simulink model "autonomy1_first_run"  (R2018a)
settings: Solver=VariableStepAuto  StartTime=0.0  StopTime=inf  RelTol=1e-3
InitFcn:
  | run('initArena.m')
undefined symbols (not defined in the file): allObstacles, endPt, wall
settings Model: SnapshotBufferSize=20  SnapshotInterval=1  Creator=alex  LastModifiedBy=alex

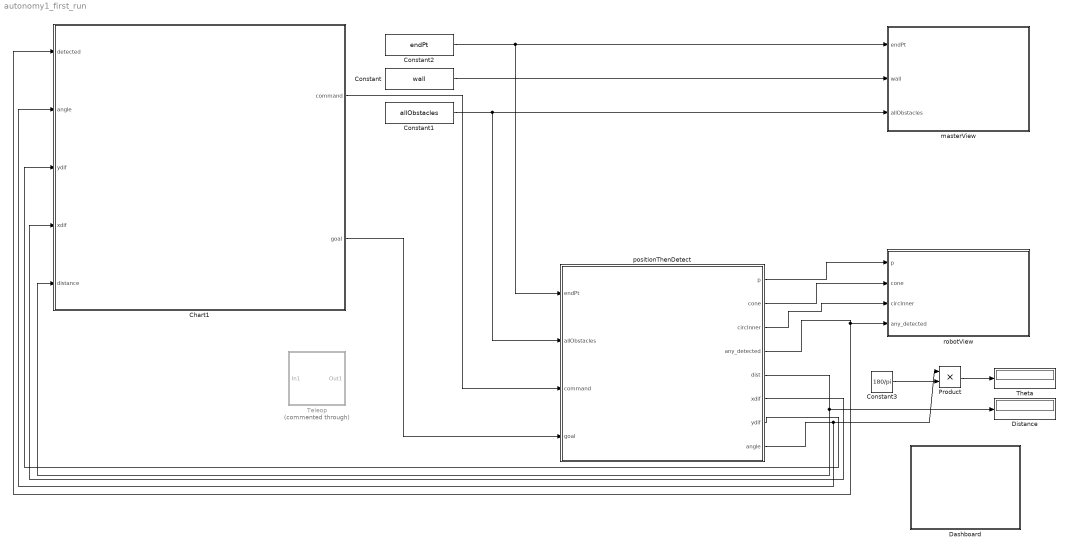
== system autonomy1_first_run ==
  Chart1 : Stateflow chart  TreatAsAtomicUnit=on
  Constant : Constant  Value=wall
  Constant1 : Constant  Value=allObstacles
  Constant2 : Constant  Value=endPt
  Constant3 : Constant  Value=180/pi
  Dashboard : Subsystem
  "Distance " : Display
  Product : Product
  "Teleop " : Subsystem  Commented=through
  Theta : Display
  masterView : MATLAB Function  TreatAsAtomicUnit=on
  positionThenDetect : MATLAB Function  TreatAsAtomicUnit=on
  robotView : MATLAB Function  TreatAsAtomicUnit=on
  wires:
  Constant/1 -> masterView/2(wall)
  Constant1/1 -> positionThenDetect/2(allObstacles), masterView/3(allObstacles)
  Chart1/1(command) -> positionThenDetect/3(command)
  positionThenDetect/4(any_detected) -> robotView/4(any_detected), Chart1/1(detected)
  Constant2/1 -> positionThenDetect/1(endPt), masterView/1(endPt)
  Constant3/1 -> Product/2
  positionThenDetect/8(angle) -> Chart1/2(angle), Product/1
  Product/1 -> Theta/1
  positionThenDetect/5(dist) -> Chart1/5(distance), "Distance "/1
  positionThenDetect/6(xdif) -> Chart1/4(xdif)
  positionThenDetect/7(ydif) -> Chart1/3(ydif)
  positionThenDetect/2(cone) -> robotView/2(cone)
  positionThenDetect/3(circInner) -> robotView/3(circInner)
  Chart1/2(goal) -> positionThenDetect/4(goal)
  positionThenDetect/1(p) -> robotView/1(p)

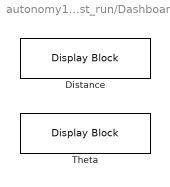
== system autonomy1_first_run/Dashboard ==
  Distance : DisplayBlock  WebBlockId=70  LabelPosition=Hide
  "Theta " : DisplayBlock  WebBlockId=71  LabelPosition=Hide

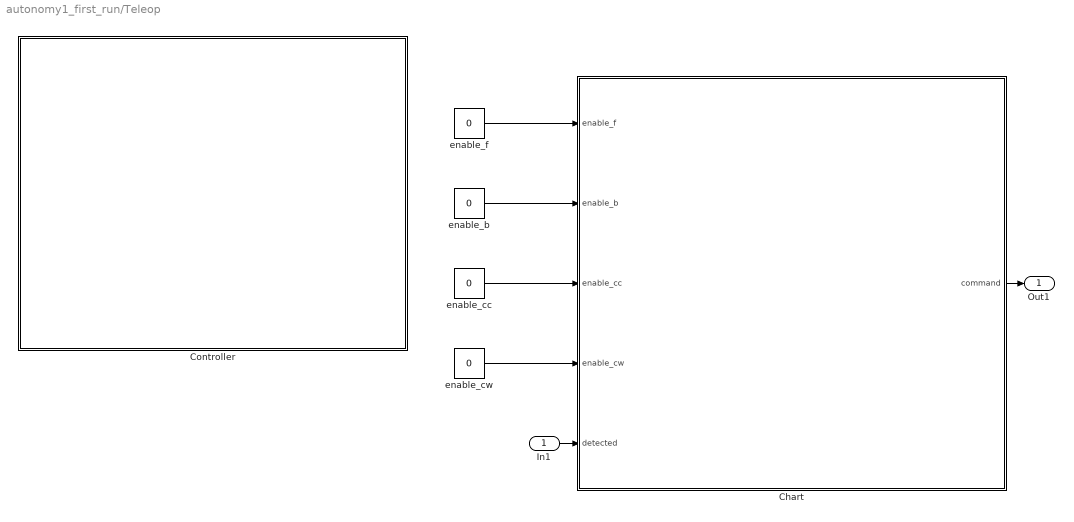
== system autonomy1_first_run/Teleop  ==
  In1 : Inport
  Chart : Stateflow chart  TreatAsAtomicUnit=on
  Controller : Subsystem
  "enable_b " : Constant  Value=0
  "enable_cc " : Constant  Value=0
  "enable_cw " : Constant  Value=0
  "enable_f " : Constant  Value=0
  Out1 : Outport
  wires:
  Chart/1(command) -> Out1/1
  "enable_cw "/1 -> Chart/4(enable_cw)
  "enable_cc "/1 -> Chart/3(enable_cc)
  "enable_b "/1 -> Chart/2(enable_b)
  In1/1 -> Chart/5(detected)
  "enable_f "/1 -> Chart/1(enable_f)

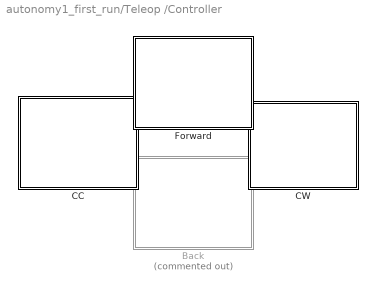
== system autonomy1_first_run/Teleop /Controller ==
  Back : Subsystem  Commented=on  DialogController=hmiCreateDDGDialog  IsWebBlock=on  mask(MWDashboardBlock){webBlockId=1a5e94ef-030e-49cd-b944-b929b04abc70, webBlockType=pushbutton, ShowInLibBrwoser=on, ShowInitialText=on, HMISrcModelName=autonomy1_first_run}
      mask prompts: webBlockId "WebBlock Id"; webBlockType "WebBlock Type"; HMISrcModelName "Source Model"
      mask help: SimulinkHMI:dialogs:PushButtonDialogDesc
      mask Help: helpview([docroot '/mapfiles/simulink.map'], 'hmi_push_button')
      mask Display:
      | model = bdroot(gcb);
      | if strcmp(get_param(model,'BlockDiagramType'), 'library')
      |     image([(matlabroot) '/toolbox/simulink/hmi/icons/PushButton.png']);
      | end
  "CC " : Subsystem  DialogController=hmiCreateDDGDialog  IsWebBlock=on  mask(MWDashboardBlock){webBlockId=f6d6ee6b-2047-45ee-ab2e-570b521bf019, webBlockType=pushbutton, ShowInLibBrwoser=on, ShowInitialText=on, HMISrcModelName=autonomy1_first_run}
      mask prompts: webBlockId "WebBlock Id"; webBlockType "WebBlock Type"; HMISrcModelName "Source Model"
      mask help: SimulinkHMI:dialogs:PushButtonDialogDesc
      mask Help: helpview([docroot '/mapfiles/simulink.map'], 'hmi_push_button')
      mask Display:
      | model = bdroot(gcb);
      | if strcmp(get_param(model,'BlockDiagramType'), 'library')
      |     image([(matlabroot) '/toolbox/simulink/hmi/icons/PushButton.png']);
      | end
  "CW " : Subsystem  DialogController=hmiCreateDDGDialog  IsWebBlock=on  mask(MWDashboardBlock){webBlockId=5b3cd59d-fae2-469c-adcb-5a1af564bf62, webBlockType=pushbutton, ShowInLibBrwoser=on, ShowInitialText=on, HMISrcModelName=autonomy1_first_run}
      mask prompts: webBlockId "WebBlock Id"; webBlockType "WebBlock Type"; HMISrcModelName "Source Model"
      mask help: SimulinkHMI:dialogs:PushButtonDialogDesc
      mask Help: helpview([docroot '/mapfiles/simulink.map'], 'hmi_push_button')
      mask Display:
      | model = bdroot(gcb);
      | if strcmp(get_param(model,'BlockDiagramType'), 'library')
      |     image([(matlabroot) '/toolbox/simulink/hmi/icons/PushButton.png']);
      | end
  Forward : Subsystem  DialogController=hmiCreateDDGDialog  IsWebBlock=on  mask(MWDashboardBlock){webBlockId=418d2ee9-92ed-471b-995b-1589f387356b, webBlockType=pushbutton, ShowInLibBrwoser=on, ShowInitialText=on, HMISrcModelName=autonomy1_first_run}
      mask prompts: webBlockId "WebBlock Id"; webBlockType "WebBlock Type"; HMISrcModelName "Source Model"
      mask help: SimulinkHMI:dialogs:PushButtonDialogDesc
      mask Help: helpview([docroot '/mapfiles/simulink.map'], 'hmi_push_button')
      mask Display:
      | model = bdroot(gcb);
      | if strcmp(get_param(model,'BlockDiagramType'), 'library')
      |     image([(matlabroot) '/toolbox/simulink/hmi/icons/PushButton.png']);
      | end

== system autonomy1_first_run/Teleop /Controller/Back ==

== system autonomy1_first_run/Teleop /Controller/CC  ==

== system autonomy1_first_run/Teleop /Controller/CW  ==

== system autonomy1_first_run/Teleop /Controller/Forward ==

== stateflow chart autonomy1_first_run/Chart1 ==
  settings: stateMachineType=MOORE_MACHINE
  state diversion
    state turn_until_clear
      command = 4
    state forward_diversion
      command = 1
    state turn_opposite_until_touch
      command = 3
    forward_diversion -> turn_until_clear [order 2] : [detected == 1]
    turn_until_clear -> forward_diversion [order 2] : [detected == 0]
    turn_opposite_until_touch -> turn_until_clear [order 2] : [detected == 1]
    forward_diversion -> turn_opposite_until_touch [order 3]
  state ideal_path
    state forward_ideal_path
      command = 1
    state turn_to_ideal
      command = 3
    forward_ideal_path -> turn_to_ideal [order 3]
  state start
    goal = [25 30]
  state arrive_mining_zone
    state arrived_mining_area
      command = 0
  turn_until_clear -> (junction 183) [order 1]
  (junction 206) -> (junction 211) [order 2] : [[(xdif < 0 & ydif > 0) | (xdif < 0 & ydif < 0)]]
  (junction 211) -> (junction 161) : [(angle < pi & angle > pi-pi/128) | (angle > -pi & angle < -pi+pi/128)]
  (junction 161) -> turn_until_clear [order 2]
  (junction 183) -> (junction 206)
  (junction 209) -> (junction 161) : [(angle > -pi/128 & angle < pi/128)]
  (junction 206) -> (junction 209) [order 1] : [(xdif > 0 & ydif > 0) | (xdif > 0 & ydif < 0)]
  forward_ideal_path -> (junction 183) [order 2]
  turn_to_ideal -> (junction 183)
  turn_opposite_until_touch -> (junction 183) [order 1]
  (junction 161) -> forward_ideal_path [order 1] : [detected == 0]
  forward_ideal_path -> (junction 200) [order 1]
  start -> turn_to_ideal
  forward_diversion -> (junction 200) [order 1]
  (junction 200) -> arrived_mining_area : [distance < 3]
  (default) -> start
  data: command output; detected input; angle input; ydif input; xdif input; distance input; goal output

== matlab function autonomy1_first_run/positionThenDetect ==
  data: p output size=[5 2]; cone output size=[4 3]; circInner output size=[2 100]; endPt input; allObstacles input; command input; any_detected output size=1; dist output size=1; xdif output size=1; ydif output size=1; angle output size=1; goal input
function [p, cone, circInner, any_detected, dist, xdif, ydif, angle] = positionThenDetect(endPt, allObstacles, command, goal)
    persistent xpos ypos theta occupancyMap
    xmax = 57; % Physical wall just outside these distances 
    ymax = 36; 
    
    % Define start location
    if isempty(xpos)
        occupancyMap = logical(zeros(ymax, xmax));
        xpos = 25;
        ypos = 3;
        theta = pi/2;
    end
        
    % Robot specifications 
    botRadius = 0.5; % Used for graphic circle and Dstar inflation 
    coneDepth = 3;
    speed = 0.5;
    turnSpeed = pi/128;

    % Radius of robot vision and representing circles 
    r = sqrt(botRadius^2+(2*coneDepth^2)-2*botRadius*sqrt(2*coneDepth^2)*cos(135*pi/180));
    t = linspace(-pi,pi);
    xc = [r*cos(t); botRadius*cos(t)];
    yc = [-r*sin(t); -botRadius*sin(t)];

    % Update position and rotation based on command 
    if command == 1 % forward
        xpos = xpos + speed*cos(theta);
        ypos = ypos + speed*sin(theta);
    elseif command == 2 % back
        xpos = xpos - speed*cos(theta);
        ypos = ypos - speed*sin(theta);
    elseif command == 3 % counter clockwise
        theta = theta + turnSpeed;
    elseif command == 4 % clockwise 
        theta = theta - turnSpeed;
    end

    % Calculate rotated cone around origin 
    thigh = theta + asin(coneDepth/r);
    tlow = thigh-2*asin(coneDepth/r);
    x = [botRadius*cos(theta) r*cos(thigh) r*cos(tlow) botRadius*cos(theta)];
    y = [botRadius*sin(theta) r*sin(thigh) r*sin(tlow) botRadius*sin(theta)];
    z = zeros(1,4);
    rotated_cone = fliplr(rot90(vertcat(x,y,z),3));
        
    % Translate cone to new position 
    cone = rotated_cone;
    cone(:,1) = rotated_cone(:,1) + xpos;
    cone(:,2) = rotated_cone(:,2) + ypos;
    cone(:,3) = rotated_cone(:,3);
    
    % Translate circle to new position 
    circInner = zeros(2, length(t));
    circInner(1,:) = xc(2,:) + xpos;
    circInner(2,:) = yc(2,:) + ypos;

    % Check if obstacle is in vision cone 
    detected = detectRotated(allObstacles, cone);
  
    % Create a list of obstacles that are detected 
    allObstX = allObstacles(:,1);
    allObstY = allObstacles(:,2);
    if (detected ~= 0)
        x = allObstX(detected==1);
        y = allObstY(detected==1);

        % Convert list of x,y coordinates to occupany map 
        occupancyMapNew = createOccupancyMap(x, y, xmax, ymax);
        occupancyMap = occupancyMap | occupancyMapNew;
    end

    % Get new path based on last map update 
    p = updatePath(occupancyMap, goal, xpos, ypos, 0);
   
    % Indicate if any obstacles are detected 
    any_detected = double(any(detected(:)));
    
    % Calculate intantaneous angle/dist between current and ideal orientation 
    angle = degFromPath(endPt, xpos, ypos, theta); 
    [dist, xdif, ydif] = distFromPath(endPt, xpos, ypos);
end

== stateflow chart autonomy1_first_run/Teleop /Chart ==
  settings: stateMachineType=MOORE_MACHINE
  state no_input
    command = 0
  state check_detected
  state back
    command = 2
  state counter_clockwise
    command = 3
  state clockwise
    command = 4
  state forward
    command = 1
  (default) -> no_input
  no_input -> check_detected [order 1] : [enable_f == 1]
  forward -> no_input [order 1] : [enable_f == 0]
  check_detected -> no_input [order 2] : [detected==1]
  no_input -> back [order 4] : [enable_b ==1]
  back -> no_input : [enable_b== 0]
  no_input -> counter_clockwise [order 3] : [enable_cc == 1]
  counter_clockwise -> no_input : [enable_cc == 0]
  no_input -> clockwise [order 2] : [enable_cw == 1]
  clockwise -> no_input : [enable_cw == 0]
  forward -> check_detected [order 2] : [detected==1]
  check_detected -> forward [order 1] : [detected==0]
  data: enable_f input; enable_b input; enable_cc input; enable_cw input; command output; detected input

== matlab function autonomy1_first_run/masterView ==
  data: endPt input; wall input; allObstacles input
function masterView(endPt, wall, allObstacles)
    % Visualize data
    plot(wall(:,1), wall(:,2), 'r-');
    hold on 
    grid on
    grid minor
    xlim([0 58]);
    ylim([0 37]);
    xlabel('Field Width (x10 cm)')
    ylabel('Field Height (x10 cm)')
    title('2D Mining Robot Simulation')
    plot(allObstacles(:,1), allObstacles(:,2), 'ks');
    plot(endPt(1), endPt(2), 'g*');
end

== matlab function autonomy1_first_run/robotView ==
  data: p input; cone input; circInner input; any_detected input
function robotView(p, cone, circInner, any_detected)
    if any_detected
        coneColor = 'r';
    else
        coneColor = 'k';
    end
    
    coneFig = plot(cone(:,1),cone(:,2), coneColor);
    circOFig = plot(circInner(1,:),circInner(2,:));
    plot(p(:,1), p(:,2), 'k*');
    set([coneFig circOFig],'LineWidth', 1)
    hold off
end
